simulink subsystem "Medium_Motor_ThorneFleissner"  (R2020b)
settings: Solver=VariableStepAuto  StartTime=0.0  StopTime=10.0  RelTol=1e-3
libraries: simulink_extras x1
settings Model: Creator=rthom  LastModifiedBy=rthom

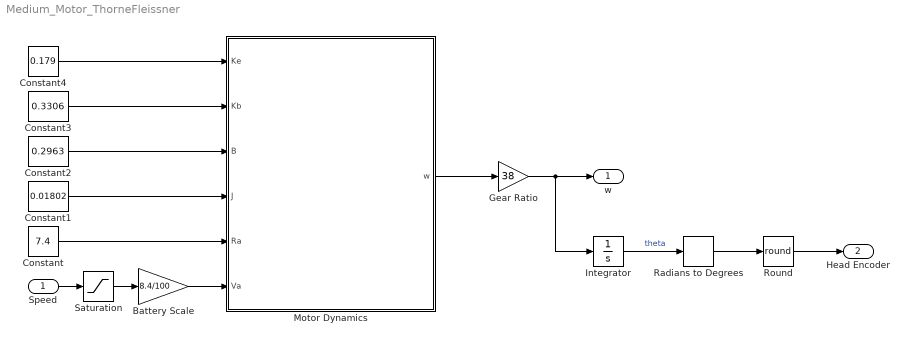
== system Medium_Motor_ThorneFleissner ==
  Speed : Inport
  Battery Scale : Gain  Gain=8.4/100
  Constant : Constant  Value=7.4
  Constant1 : Constant  Value=0.01802
  Constant2 : Constant  Value=0.2963
  Constant3 : Constant  Value=0.3306
  Constant4 : Constant  Value=0.179
  Gear Ratio : Gain  Gain=38
  Integrator : Integrator
  Motor Dynamics : Subsystem
  Radians to Degrees : simulink_extras/Transformations/Radians to Degrees
  Round : Rounding  Operator=round
  Saturation : Saturate  UpperLimit=100  LowerLimit=-100
  w : Outport
  Head Encoder : Outport  Port=2
  wires:
  Constant/1 -> Motor Dynamics/5(Ra)
  Constant1/1 -> Motor Dynamics/4(J)
  Constant2/1 -> Motor Dynamics/3(B)
  Constant3/1 -> Motor Dynamics/2(Kb)
  Constant4/1 -> Motor Dynamics/1(Ke)
  Motor Dynamics/1(w) -> Gear Ratio/1
  Gear Ratio/1 -> w/1, Integrator/1
  Battery Scale/1 -> Motor Dynamics/6(Va)
  Speed/1 -> Saturation/1
  Saturation/1 -> Battery Scale/1
  Integrator/1 -> Radians to Degrees/1  "theta"
  Radians to Degrees/1 -> Round/1
  Round/1 -> Head Encoder/1

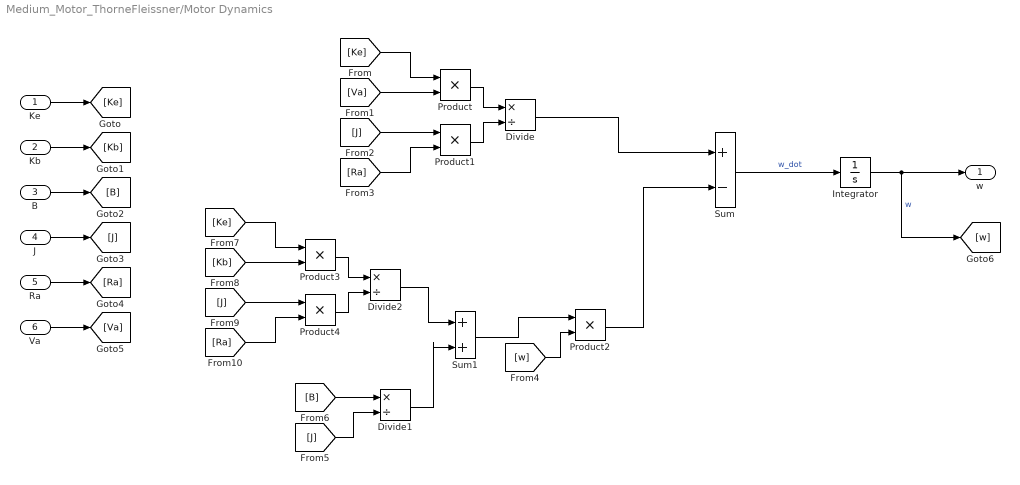
== system Medium_Motor_ThorneFleissner/Motor Dynamics ==
  Ke : Inport
  Kb : Inport  Port=2
  B : Inport  Port=3
  J : Inport  Port=4
  Ra : Inport  Port=5
  Va : Inport  Port=6
  Divide : Product  Inputs=*/
  Divide1 : Product  Inputs=*/
  Divide2 : Product  Inputs=*/
  Integrator : Integrator
  Product{,1..4} (5 alike) : Product
  Sum : Sum  Inputs=+-
  Sum1 : Sum
  w : Outport
  wires:
  Divide2/1 -> Sum1/1
  [Kb] -> Product3/2
  [Ke] -> Product3/1
  [J] -> Product4/1
  Product4/1 -> Divide2/2
  Product3/1 -> Divide2/1
  [Ra] -> Product4/2
  [B] -> Divide1/1
  [J] -> Divide1/2
  Divide1/1 -> Sum1/2
  Sum1/1 -> Product2/1
  [w] -> Product2/2
  Product2/1 -> Sum/2
  Divide/1 -> Sum/1
  [Ra] -> Product1/2
  [J] -> Product1/1
  [Va] -> Product/2
  [Ke] -> Product/1
  Product1/1 -> Divide/2
  Product/1 -> Divide/1
  Va/1 -> [Va]
  Ra/1 -> [Ra]
  J/1 -> [J]
  B/1 -> [B]
  Kb/1 -> [Kb]
  Ke/1 -> [Ke]
  Sum/1 -> Integrator/1  "w_dot"
  Integrator/1 -> w/1, [w]  "w"
